simulink model "SEM_MBD_Bike_CMG_2017b"  (R2017b)
settings: Solver=FixedStepAuto  StartTime=0.0  StopTime=Tend  FixedStep=1e-3  MaxStep=0.01  RelTol=1e-4  AbsTol=1e-5  EnableMultiTasking=on
PreLoadFcn:
  | addpath(genpath('SM_Contact'))
  | addpath('include')
InitFcn:
  | MBD_Intfn
model workspace (MATLAB code in the model file):
  | whl.rad = 0.025;
  | whl.thickness = 0.005;
  | 
  | axle.length = 0.2;
  | axle.radius = 0.005;
  | platform.radius = 0.15;
  | platform.thickness = 0.005;
  | platform.offset = -0.01;
  | 
  | bumper.rad = platform.offset+whl.rad;
  | 
  | 
  | 
  | table.length = 1;
  | table.thickness = 0.01;
  | tableWhl.contact.k = 1e3;
  | tableWhl.contact.b = 1e2;
  | 
  | steel.density = 8000; %kg/m^3
  | 
  | start_pos.x = -0.2;
  | start_pos.y = 0.2;
  | 
  | l_whl_trq = [0 0 0 0.5 0 0 0 -0.5 1.0 0 0 0 -1.0 0.5 0 0 0 -0.5 -1.5 0 0 0 1.5].'*0.0005;
  | r_whl_trq = [0 0 0 2.0 0 0 0 -2.0 1.0 0 0 0 -1.0 1.0 0 0 0 -1.0 -1.5 0 0 0 1.5].'*0.0005;
values from neighbouring files (symbols this model uses):
  Dfw = 0.6    [MBD_Intfn.m]
  Drw = 0.6    [MBD_Intfn.m]
  followerCameraX = -1.5    [MBD_Intfn.m]
  followerCameraY = 0.5    [MBD_Intfn.m]
  followerCameraZ = -3    [MBD_Intfn.m]
  H = 1/2    (= 0.5)    [MBD_Intfn.m]
  IntG = 70    [MBD_Intfn.m]
  IntP = 0    [MBD_Intfn.m]
  isoCameraAimX = (1/2)*L    (= 1)    [MBD_Intfn.m]
  isoCameraX = -3.1    [MBD_Intfn.m]
  isoCameraY = 3.5    [MBD_Intfn.m]
  isoCameraZ = 1.5    [MBD_Intfn.m]
  Kdelta = -2.5    [MBD_Intfn.m]
  Kdeltadot = -5    [MBD_Intfn.m]
  Kphi = -60    [MBD_Intfn.m]
  Kphidot = -6    [MBD_Intfn.m]
  Ktheta = 0.1    [MBD_Intfn.m]
  Kthetadot = -5    [MBD_Intfn.m]
  Kv = -2.69    [MBD_Intfn.m]
  L = 2    [MBD_Intfn.m]
  Ldelta = 15    [MBD_Intfn.m]
  M = 10    [MBD_Intfn.m]
  MF = 1    [MBD_Intfn.m]
  Mf = 2    [MBD_Intfn.m]
  MR = 1    [MBD_Intfn.m]
  Nf = 5000    [MBD_Intfn.m]
  Rdelta = 0    [MBD_Intfn.m]
  refphi = 0    [MBD_Intfn.m]
  reftheta = 0    [MBD_Intfn.m]
  Rf = 0.2    [MBD_Intfn.m]
  Switch = 0    [MBD_Intfn.m]
  T = 0.05    [MBD_Intfn.m]
  tdl = 10    [MBD_Intfn.m]
  tdr = 1    [MBD_Intfn.m]
  Tend = 35    [MBD_Intfn.m]
  Tf = 0.3/5    (= 0.06)    [MBD_Intfn.m]
  topCameraX = -4.5    [MBD_Intfn.m]
  topCameraY = 0    [MBD_Intfn.m]
  topCameraZ = -0.5    [MBD_Intfn.m]
  tpdl = 10    [MBD_Intfn.m]
  tpdr = 1    [MBD_Intfn.m]
  v = 5    [MBD_Intfn.m]
undefined symbols (not defined in the file or in its folder): Floor, X, Y, Z
libraries: sm_lib x52, nesl_utility x41, Parts_Lib x4, Contact_Forces_Lib x4, simulink x2, fl_lib x1
(part 1 of 3)
Description:
  | A simulator for a simplified bicycle model including a CMG
  | 
  | By:
  | Dinesh Thirumurugan
  | Bhavesh Kataria
  | Allauddin Shaikh
  | Alen Turnwald
settings Model: Creator=smiller  LastModifiedBy=Alen
settings SolverCC: PositivePriorityOrder=on  AutoInsertRateTranBlk=on
settings DataIOCC: MaxDataPoints=15000  SaveFormat=Array  SignalLoggingName=logsout_Robot_2_Whl
settings OptimizationCC: EnhancedBackFolding=on  PassReuseOutputArgsThreshold=0  MaxStackSize=64  OptimizeBlockOrder=speed  DifferentSizesBufferReuse=on
settings DebuggingCC: SolverPrmCheckMsg=warning  ParameterTunabilityLossMsg=error  UnconnectedInputMsg=none  UnconnectedOutputMsg=none  AllowSymbolicDim=off  SFUnexpectedBacktrackingDiag=warning  SFNoUnconditionalDefaultTransitionDiag=warning  SFExecutionAtInitializationDiag=none
settings HardwareCC: ProdBitPerPointer=32  ProdBitPerSizeT=32  ProdBitPerPtrDiffT=32  ProdLargestAtomicInteger=Long  ProdLargestAtomicFloat=Double  ProdWordSize=32  ProdHWDeviceType=ARM Compatible->ARM Cortex  UseEmbeddedCoderFeatures=off
settings ModelReferenceCC: PropagateSignalLabelsOutOfModel=off
settings SFSimCC: MATLABDynamicMemAlloc=off
settings RTWCC: SystemTargetFile=ert.tlc  HardwareBoard=Raspberry Pi  TemplateMakefile=ert_default_tmf  GenerateReport=on  Toolchain=GNU GCC Raspberry Pi  BuildConfiguration=Faster Runs  LaunchReport=on
settings CodeAppCC: ForceParamTrailComments=on  OperatorAnnotations=on
settings ERTTargetCC: ERTCustomFileBanners=off  SupportContinuousTime=on  SupportNonInlinedSFcns=on  RemoveResetFunc=off  SupportVariableSizeSignals=on  ModelStepFunctionPrototypeControlCompliant=off
settings ConfigComp: CovMetricSettings=dw  CovHtmlReporting=on  CovSaveCumulativeToWorkspaceVar=on  CovSaveSingleToWorkspaceVar=on  CovExternalEMLEnable=off  CovSFcnEnable=off
settings SimscapeCC: SimscapeNormalizeSystem=off  SimscapeLogType=all  SimscapeLogSimulationStatistics=on  SimscapeLogName=simlog_Robot_2_Whl  SimscapeLogDataHistory=15000
settings ConfigurationSet: Description=SimMechanics 2G
settings DiagnosticsConfigSet: SimMechanicsRigidlyBoundBlock=none
settings ExplorerConfigSet: InternalSimMechanicsExplorerSettings="<ExplorerConfiguration><canonicalview>default</canonicalview><AnimationSetting><BasePlaybackSpeed>1.0</BasePlaybackSpeed><PlaybackSpeedFactor>1.0</PlaybackSpeedFactor></AnimationSetting><TilePanel><TileInfo><Tiles Columns=\"2\" Count=\"2\" Rows=\"1\"><Column Weight=\"0.5\"/><Column Weight=\"0.5\"/><Row Weight=\"1\"/><Tile Height=\"1\" Width=\"1\" X=\"0\" Y=\"0\"/><Tile Height=\"1\" Width=\"1\" X=\"1\" Y=\"0\"/></Tiles></TileInfo><SceneInfo><SceneViewer><BGColor><R>0.913725495338439941</R><G>0.952941179275512695</G><B>0.952941179275512695</B></BGColor><Camera><DoPerspective>on</DoPerspective><Position><X>19.7957692472944586</X><Y>-22.1490524136403373</Y><Z>1.79876643323261254</Z></Position><Center><X>22.8384549439588795</X><Y>-22.2465600466053246</Y><Z>0.30459240962381362</Z></Center><Up><X>0</X><Y>0</Y><Z>1</Z></Up><ViewLimDist>1</ViewLimDist><YLim>0.466307658154998583</YLim><XLim>0.393531318442946809</XLim></Camera></SceneViewer><SceneViewer><BGColor><R>0.913725495338439941</R><G>0.952941179275512695</G><B>0.952941179275512695</B></BGColor><Camera><DoPerspective>on</DoPerspective><Position><X>22.3361107324775219</X><Y>-22.2651355831809319</Y><Z>4.80429298217662559</Z></Position><Center><X>22.8384549439588795</X><Y>-22.2465600466053246</Y><Z>0.30459240962381362</Z></Center><Up><X>0</X><Y>0</Y><Z>1</Z></Up><ViewLimDist>1</ViewLimDist><YLim>0.466307658154998583</YLim><XLim>0.393531318442946809</XLim></Camera></SceneViewer></SceneInfo></TilePanel><MechEditorPanel><Cameras><Camera><Id>Camera1</Id><Value><Name>Follower Camera</Name><NativeCamera><PositionTrackingFeature>x1.Frame.Cameras.Follower_Camera_Transform.F</PositionTrackingFeature><CenterTrackingFeature>x1.Frame.Frame.R</CenterTrackingFeature><UpVectorTrackingFeature>x1.World_Frame.W</UpVectorTrackingFeature><CenterTrackingOrigin>on</CenterTrackingOrigin><UpVectorTrackingDirection>+Z</UpVectorTrackingDirection></NativeCamera></Value></Camera><Camera><Id>Camera2</Id><Value><Name>Top Camera</Name><NativeCamera><PositionTrackingFeature>x1.Frame.Cameras.Follower_Camera_Transform1.F</PositionTrackingFeature><CenterTrackingFeature>x1.Frame.Frame.R</CenterTrackingFeature><UpVectorTrackingFeature>x1.World_Frame.W</UpVectorTrackingFeature><CenterTrackingOrigin>on</CenterTrackingOrigin><UpVectorTrackingDirection>+Z</UpVectorTrackingDirection></NativeCamera></Value></Camera></Cameras><GfxPanelCameraMap><MapElement CameraMLId=\"Camera1\" GfxPanelIndex=\"0\"/><MapElement CameraMLId=\"Camera2\" GfxPanelIndex=\"1\"/></GfxPanelCameraMap><VideoCreator><PlaybackSpeedRatio>1.0</PlaybackSpeedRatio><FrameRate>30</FrameRate><VideoFormat>Motion JPEG AVI</VideoFormat><FrameSize>[800 600]</FrameSize></VideoCreator></MechEditorPanel></ExplorerConfiguration>"

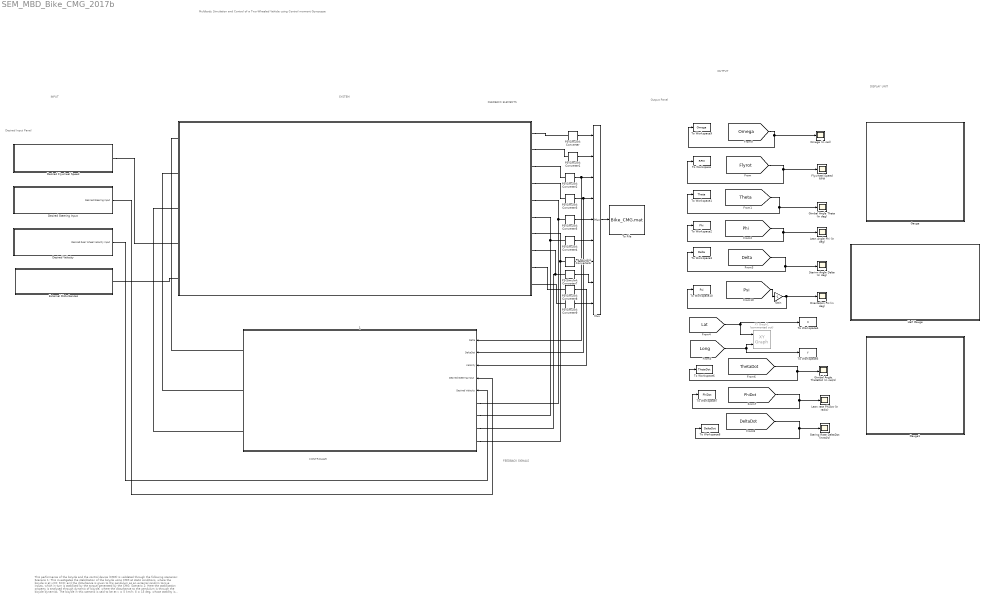
== system SEM_MBD_Bike_CMG_2017b ==
  note: Multibody Simulation and Control of a Two-Wheeled Vehicle using Control moment Gyroscope
  note: This performance of the bicycle and the control device (CMG) is validated through the following scenarios:
      |
      | Scenario 1: This investigates the stabilization of the bicycle using CMG at static conditions, where the bicycle is at v=0; δ=0; and the disturbance is given to the pendulum as an external random torque inputs, which in turn is stabilized by the torque generated by the CMG.
      |
      | Scenario 2: Here the stabilization property is analysed through dynamic of bicycle, where the disturbance to the pendulum is through the bicycle dynamics. The bicycle in this scenario is said to be at v = 5 km/h; δ = 15 deg, whose stability is analysed through the inverted pendulum which in turn is stabilized by the CMG.
      |
      | Scenario 3: The general behaviour of the bicycle dynamics is investigated in this scenario, here the control device is kept completely inactive and the pendulum is put at completely downward resting position. The bicycle is give a velocity v>0; and steering δ>0 for a specific time period to inspect the forces generated while cornering to produce a leaning behaviour by the pendulum approximating to that of the bicycle behaviour.
  note: Output Panel
  note: INPUT
  note: Desired Input Panel
  note: SYSTEM
  note: OUTPUT
  note: FEEDBACK SIGNALS
  note: CONTROLLER
  note: FEEDBACK ELEMENTS
  note: DISPLAY UNIT
  " " : Subsystem  mask(Controllers Parameters){Kphi=Kphi, Kphidot=Kphidot, Ktheta=Ktheta, Kthetadot=Kthetadot, refphi=refphi, reftheta=reftheta, Kdelta=Kdelta, Kdeltadot=Kdeltadot, Kv=Kv}
      mask prompts: Kphi "Proportional Gain Kφ"; Kphidot "Derivative Gain Kφ'"; Ktheta "Proptional Gain Kθ"; Kthetadot "Derivative Gain Kθ'"; refphi "Reference angle for pendulum (in deg)"; reftheta "Referance gimbal precision angle"; Kdelta "Proportional Gain Kδ"; Kdeltadot "Derivative Gain Kδ'"; Kv "Proportional Gain Kv"
      mask help:
      | PD Controller for Bicycle Stability:
      |
      | τ(θ) = −Kφ*(φ − φd) − Kφ˙*(φ˙) − Kθ*(θ − θd) − K˙θ*(˙θ).
      |
      | --------------------------------------------------------------------------------------------------------------------------------------------------------------
      | PD Controller for Steering:
      |
      | τ(δ) = −Kδ*(δ − δd) − K˙δ*(˙δ)
      |
      | --------------------------------------------------------------------------------------------------------------------------------------------------------------
      | PD Controller for Rear Wheel Torque:
      |
      | τ(v) = −Kv*(v − vd)
      mask Display: image('RPI.png')
  " 1" : Subsystem  mask(Controllers Parameters){Kphi=Kphi, Kphidot=Kphidot, Ktheta=Ktheta, Kthetadot=Kthetadot, refphi=refphi, reftheta=reftheta, Kdelta=Kdelta, Kdeltadot=Kdeltadot, Kv=Kv}
      mask prompts: Kphi "Proportional Gain Kφ"; Kphidot "Derivative Gain Kφ'"; Ktheta "Proptional Gain Kθ"; Kthetadot "Derivative Gain Kθ'"; refphi "Reference angle for pendulum (in deg)"; reftheta "Referance gimbal precision angle"; Kdelta "Proportional Gain Kδ"; Kdeltadot "Derivative Gain Kδ'"; Kv "Proportional Gain Kv"
      mask help:
      | PD Controller for Bicycle Stability:
      |
      | τ(θ) = −Kφ*(φ − φd) − Kφ˙*(φ˙) − Kθ*(θ − θd) − K˙θ*(˙θ).
      |
      | --------------------------------------------------------------------------------------------------------------------------------------------------------------
      | PD Controller for Steering:
      |
      | τ(δ) = −Kδ*(δ − δd) − K˙δ*(˙δ)
      |
      | --------------------------------------------------------------------------------------------------------------------------------------------------------------
      | PD Controller for Rear Wheel Torque:
      |
      | τ(v) = −Kv*(v − vd)
      mask Display: image('RPI.png')
  "           " : Subsystem  mask(Parameters of bicycle with CMG){cyl_dia_R=Drw, cyl_dia_F=Dfw, cyl_thickness=T, cyl_mass_R=MR, cyl_mass_F=MF, BaseL=L, Bikemass=M, Fly_R=Rf, Fly_T=Tf, Fly_M=Mf, CMG_H=H, IntP=IntP, IntG=IntG}
      mask prompts: cyl_dia_R "Diameter of rear wheel (in m)"; cyl_dia_F "Diameter of front wheel (in m)"; cyl_thickness "Wheel thickness (in m)"; cyl_mass_R "Mass of the rear wheel (in kg)"; cyl_mass_F "Mass of the front wheel (in kg)"; BaseL "Wheelbase (in m)"; Bikemass "Mass of the bicycle (frame included) (in kg)"; Fly_R "Radius of flywheel (in m)"; Fly_T "Thickness of flywheel (in m)"; Fly_M "Mass of flywheel (in kg)"; CMG_H "Height of the CMG (in m)"; IntP "Initial position of pendulum (in deg)"; IntG "Initial position of the gimbal (in deg)"
      mask help:
      | The given parameters are used for model creation.
      |
      | ------------------------------------------------------------------------------------------------------------------------------------------------------------------
      mask Display: image('Bike_CSs.jpg')
  Desired Flywheel Speed : Subsystem  mask(Flywheel Rotation Speed){w=Nf}
      mask prompts: w "Flywheel Speed (RPM)"
      mask help: Omega (RPM)
  Desired Steering Input : Subsystem  mask(Desired Steering Input){t=Tend, delta_L=Ldelta, l_t=tpdl, Lt=tdl, delta_R=Rdelta, r_t=tpdr, Rt=tdr}
      mask prompts: t "Total Time Duration (in sec)"; delta_L "Left Steering Angle (in deg)"; l_t "Phase delay - Left Steering (in sec)"; Lt "Duration for Left Steering (in sec)"; delta_R "Right Steering Angle (in deg)"; r_t "Phase delay - Right Steering (in sec)"; Rt "Duration for Right Steering (in sec)"
      mask help:
      | This block helps to build a steering profile for the bicycle to follow.
      |
      | --------------------------------------------------------------------------------------------------------------------------------------------------------------
      | Total Time Duration  = Total time duration for simulation signal (in sec)
      |
      | %Left steering inputs
      | Left Steering Angle (in deg) = Left steering angle (in deg) defines the angle input requried for left steering
      | Phase delay - Left Steering (in sec) = Phase delay for left steering (in sec) defines the time duration after which the left steering angle input should be achived
      | Duration for Left Steering (in sec) = Duration for the left steering (in sec) defines the duration for which the left steering signal should be active
      |
      | %Right steering inputs
      | Right Steering Angle (in deg) = Right steering angle (in deg) defines the angle input requried for right steering
      | Phase delay - Right Steering (in sec) = Phase delay for right steering (in sec) defines the time duration after which the right steering angle input should be achived
      | Duration for Right Steering (in sec) = Duration for the right steering (in sec) defines the duration for which the right steering signal should be active
  Desired Velocity : Subsystem  mask{v=v}
      mask prompts: v "Desired Velocity (kmph)"
  External Disturbances : Subsystem  mask{Switch=Switch}
      mask prompts: Switch "External Disturbance Enable/Disable"
  Flywheel Speed RPM : Scope
  Gain : Gain  Gain=-1
  Gauge : Subsystem  DialogController=hmiCreateDDGDialog  IsWebBlock=on  mask(MWDashboardBlock){webBlockId=e0acaf17-1707-462e-bd3e-ad1907f2a35e, webBlockType=circulargauge, ShowInLibBrowser=on, ShowInitialText=on, HMISrcModelName=SEM_MBD_Bike_CMG_2017b}
      mask prompts: webBlockId "WebBlock Id"; webBlockType "WebBlock Type"; HMISrcModelName "Source Model"
      mask help: SimulinkHMI:dialogs:CircularGaugeDialogDesc
      mask Help: helpview([docroot '/mapfiles/simulink.map'], 'hmi_gauge')
      mask Display:
      | if strcmp(get_param(bdroot(gcb),'BlockDiagramType'), 'library')
      |     image([(matlabroot) '/toolbox/simulink/hmi/icons/CircularGauge.png']);
      | end
  Gauge1 : Subsystem  DialogController=hmiCreateDDGDialog  IsWebBlock=on  mask(MWDashboardBlock){webBlockId=d5ddcee6-ece7-4a8c-aff1-6e72436c5361, webBlockType=circulargauge, ShowInLibBrowser=on, ShowInitialText=on, HMISrcModelName=SEM_MBD_Bike_CMG_2017b}
      mask prompts: webBlockId "WebBlock Id"; webBlockType "WebBlock Type"; HMISrcModelName "Source Model"
      mask help: SimulinkHMI:dialogs:CircularGaugeDialogDesc
      mask Help: helpview([docroot '/mapfiles/simulink.map'], 'hmi_gauge')
      mask Display:
      | if strcmp(get_param(bdroot(gcb),'BlockDiagramType'), 'library')
      |     image([(matlabroot) '/toolbox/simulink/hmi/icons/CircularGauge.png']);
      | end
  Gimbal Angle Theta (in deg) : Scope
  Gimbal Angle ThetaDot (in rad/s) : Scope
  Half Gauge : Subsystem  DialogController=hmiCreateDDGDialog  IsWebBlock=on  mask(MWDashboardBlock){webBlockId=2bf35224-e477-42b1-a6f6-088c116ad7f4, webBlockType=semicirculargauge, ShowInLibBrowser=on, ShowInitialText=on, HMISrcModelName=SEM_MBD_Bike_CMG_2017b}
      mask prompts: webBlockId "WebBlock Id"; webBlockType "WebBlock Type"; HMISrcModelName "Source Model"
      mask help: SimulinkHMI:dialogs:SemicircularGaugeDialogDesc
      mask Help: helpview([docroot '/mapfiles/simulink.map'], 'hmi_half_gauge')
      mask Display:
      | if strcmp(get_param(bdroot(gcb),'BlockDiagramType'), 'library')
      |     image([(matlabroot) '/toolbox/simulink/hmi/icons/SemicircularGauge.png']);
      | end
  "Lean Angle Phi (in deg) " : Scope
  Lean rate PhiDot (in rad/s) : Scope
  Mux : Mux  Inputs=9
  Omega (in rad) : Scope
  Orientation Psi (in deg) : Scope
  PS-Simulink Converter : nesl_utility/PS-Simulink Converter  PhysicalDomain=network_engine_domain  SubClassName=ps_output  LeftPortType=input  RightPortType=output  PseudoPeriodic=off  Frequencies=[]  Unit=m  AffineConversion=off
  PS-Simulink Converter1 : nesl_utility/PS-Simulink Converter  PhysicalDomain=network_engine_domain  SubClassName=ps_output  LeftPortType=input  RightPortType=output  PseudoPeriodic=off  Frequencies=[]  Unit=m  AffineConversion=off
  PS-Simulink Converter{2..9} (8 alike) : nesl_utility/PS-Simulink Converter  PhysicalDomain=network_engine_domain  SubClassName=ps_output  LeftPortType=input  RightPortType=output  PseudoPeriodic=off  Frequencies=[]  Unit=1  AffineConversion=off
  Stering Angle Delta (in deg) : Scope
  Stering Rate DeltaDot (inrad/s) : Scope
  To File : ToFile  Filename=Bike_CMG.mat  MatrixName=output  SaveFormat=Timeseries
  To Workspace : ToWorkspace  VariableName=RPM  SaveFormat=Timeseries  SampleTime=-1
  To Workspace1 : ToWorkspace  VariableName=Theta  SaveFormat=Timeseries  SampleTime=-1
  To Workspace10 : ToWorkspace  VariableName=Psi  SaveFormat=Timeseries  SampleTime=-1
  To Workspace2 : ToWorkspace  VariableName=Phi  SaveFormat=Timeseries  SampleTime=-1
  To Workspace3 : ToWorkspace  VariableName=Delta  SaveFormat=Timeseries  SampleTime=-1
  To Workspace4 : ToWorkspace  VariableName=X  SaveFormat=Timeseries  SampleTime=-1
  To Workspace5 : ToWorkspace  VariableName=Y  SaveFormat=Timeseries  SampleTime=-1
  To Workspace6 : ToWorkspace  VariableName=ThetaDot  SaveFormat=Timeseries  SampleTime=-1
  To Workspace7 : ToWorkspace  VariableName=PhiDot  SaveFormat=Timeseries  SampleTime=-1
  To Workspace8 : ToWorkspace  VariableName=DeltaDot  SaveFormat=Timeseries  SampleTime=-1
  To Workspace9 : ToWorkspace  VariableName=Omega  SaveFormat=Timeseries  SampleTime=-1
  XY Graph1 : simulink/Sinks/XY Graph  Commented=on  xmin=-50  xmax=50  ymin=-50  ymax=50  st=0.5
  wires:
  [Flyrot] -> To Workspace/1, Flywheel Speed RPM/1
  [Theta] -> To Workspace1/1, Gimbal Angle Theta (in deg)/1
  [Phi] -> To Workspace2/1, "Lean Angle Phi (in deg) "/1
  [Delta] -> To Workspace3/1, Stering Angle Delta (in deg)/1
  [Lat] -> XY Graph1/1, To Workspace4/1
  [Long] -> XY Graph1/2, To Workspace5/1
  [ThetaDot] -> To Workspace6/1, Gimbal Angle ThetaDot (in rad/s)/1
  [PhiDot] -> To Workspace7/1, Lean rate PhiDot (in rad/s)/1
  [DeltaDot] -> To Workspace8/1, Stering Rate DeltaDot (inrad/s)/1
  PS-Simulink Converter7/1 -> Mux/8
  PS-Simulink Converter6/1 -> Mux/7
  PS-Simulink Converter4/1 -> Mux/6
  PS-Simulink Converter5/1 -> Mux/5
  PS-Simulink Converter1/1 -> Mux/2
  PS-Simulink Converter/1 -> Mux/1
  PS-Simulink Converter9/1 -> Mux/9
  Mux/1 -> To File/1
  PS-Simulink Converter2/1 -> " "/1(Delta), Mux/3
  PS-Simulink Converter8/1 -> " "/3(Velocity)
  PS-Simulink Converter3/1 -> " "/2(DeltaDot), Mux/4
  Desired Steering Input/1(Desired Steering Input) -> " "/4(Desired Steering Input)
  Desired Velocity/1(Desired Rear Wheel Velocity Input) -> " "/5(Desired Velocity)
  [Omega] -> To Workspace9/1, Omega (in rad)/1
  [Psi] -> Gain/1
  Gain/1 -> To Workspace10/1, Orientation Psi (in deg)/1
  connections:
  "           "/LConn1 -- PS-Simulink Converter/LConn1
  "           "/LConn2 -- PS-Simulink Converter1/LConn1
  "           "/LConn3 -- PS-Simulink Converter2/LConn1
  "           "/LConn4 -- PS-Simulink Converter3/LConn1
  "           "/LConn5 -- " "/LConn1 -- PS-Simulink Converter5/LConn1
  "           "/LConn6 -- " "/LConn2 -- PS-Simulink Converter4/LConn1
  "           "/LConn7 -- " "/LConn4 -- PS-Simulink Converter6/LConn1
  "           "/LConn8 -- " "/LConn3 -- PS-Simulink Converter7/LConn1
  "           "/LConn9 -- PS-Simulink Converter8/LConn1
  " "/RConn1 -- "           "/RConn1
  " "/RConn2 -- "           "/RConn2
  " "/RConn3 -- "           "/RConn3
  PS-Simulink Converter9/LConn1 -- "           "/LConn10
  Desired Flywheel Speed/RConn1 -- "           "/RConn4
  "           "/RConn5 -- External Disturbances/RConn1

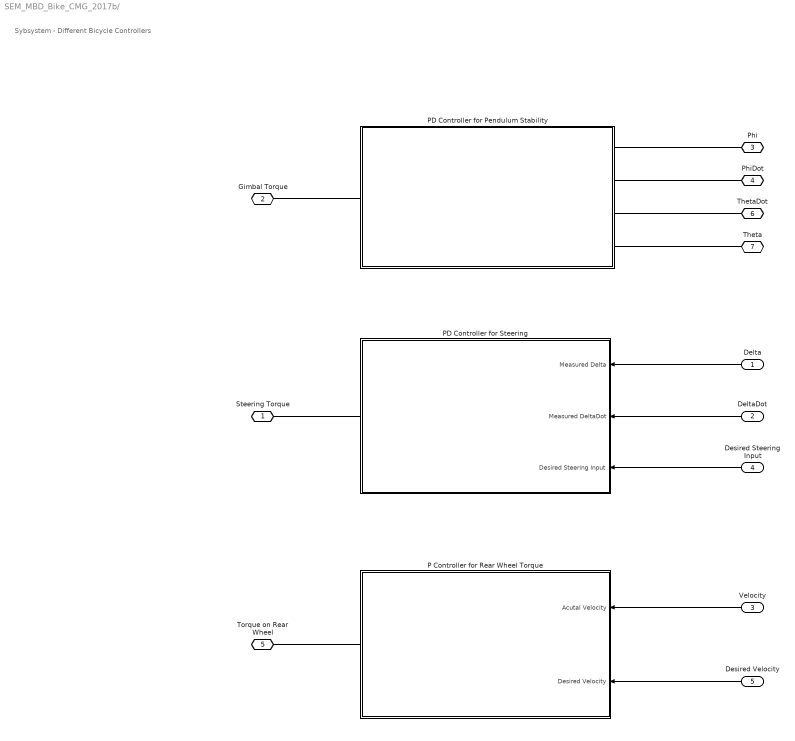
== system SEM_MBD_Bike_CMG_2017b/  ==
  note: Sybsystem - Different Bicycle Controllers
  Delta : Inport
  DeltaDot : Inport  Port=2
  Velocity : Inport  Port=3
  Desired Steering Input : Inport  Port=4
  Desired Velocity : Inport  Port=5
  "P Controller for Rear Wheel Torque " : Subsystem
  "PD Controller for Pendulum Stability " : Subsystem
  "PD Controller for Steering " : Subsystem
  Steering Torque : PMIOPort  Port=1  Side=Right
  "Gimbal Torque " : PMIOPort  Port=2  Side=Right
  Phi : PMIOPort  Port=3  Side=Left
  PhiDot : PMIOPort  Port=4  Side=Left
  Torque on Rear Wheel : PMIOPort  Port=5  Side=Right
  ThetaDot : PMIOPort  Port=6  Side=Left
  Theta : PMIOPort  Port=7  Side=Left
  wires:
  Delta/1 -> "PD Controller for Steering "/1(Measured Delta)
  Velocity/1 -> "P Controller for Rear Wheel Torque "/1(Acutal Velocity)
  DeltaDot/1 -> "PD Controller for Steering "/2(Measured DeltaDot)
  Desired Steering Input/1 -> "PD Controller for Steering "/3(Desired Steering Input)
  Desired Velocity/1 -> "P Controller for Rear Wheel Torque "/2(Desired Velocity)
  connections:
  "PD Controller for Pendulum Stability "/LConn1 -- Phi/RConn1
  "P Controller for Rear Wheel Torque "/RConn1 -- Torque on Rear Wheel/RConn1
  "PD Controller for Pendulum Stability "/LConn2 -- PhiDot/RConn1
  "PD Controller for Pendulum Stability "/LConn3 -- ThetaDot/RConn1
  "PD Controller for Steering "/RConn1 -- Steering Torque/RConn1
  "PD Controller for Pendulum Stability "/RConn1 -- "Gimbal Torque "/RConn1
  Theta/RConn1 -- "PD Controller for Pendulum Stability "/LConn4

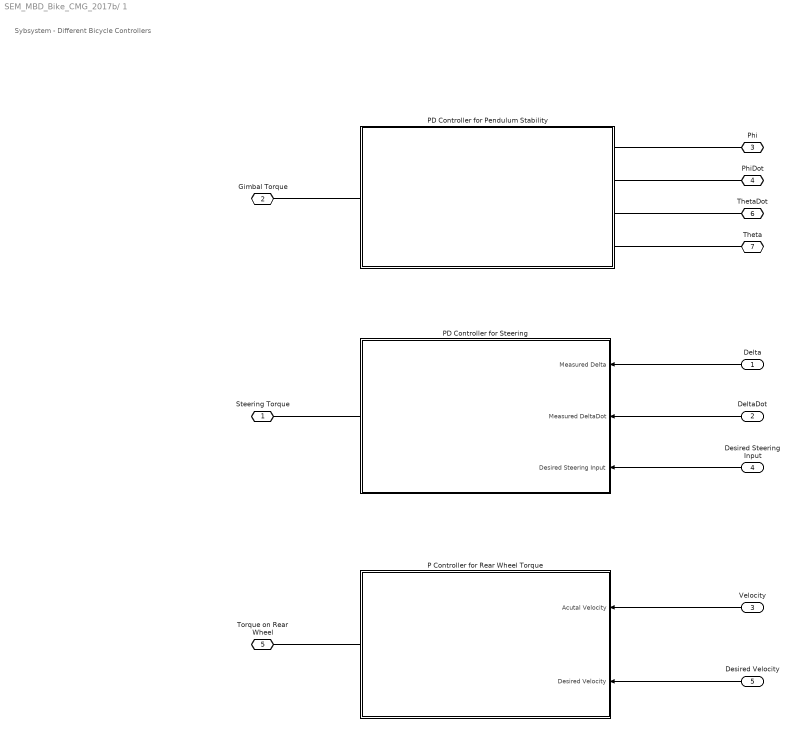
== system SEM_MBD_Bike_CMG_2017b/ 1 ==
  note: Sybsystem - Different Bicycle Controllers
  Delta : Inport
  DeltaDot : Inport  Port=2
  Velocity : Inport  Port=3
  Desired Steering Input : Inport  Port=4
  Desired Velocity : Inport  Port=5
  "P Controller for Rear Wheel Torque " : Subsystem
  "PD Controller for Pendulum Stability " : Subsystem
  "PD Controller for Steering " : Subsystem
  Steering Torque : PMIOPort  Port=1  Side=Right
  "Gimbal Torque " : PMIOPort  Port=2  Side=Right
  Phi : PMIOPort  Port=3  Side=Left
  PhiDot : PMIOPort  Port=4  Side=Left
  Torque on Rear Wheel : PMIOPort  Port=5  Side=Right
  ThetaDot : PMIOPort  Port=6  Side=Left
  Theta : PMIOPort  Port=7  Side=Left
  wires:
  Desired Velocity/1 -> "P Controller for Rear Wheel Torque "/2(Desired Velocity)
  Desired Steering Input/1 -> "PD Controller for Steering "/3(Desired Steering Input)
  DeltaDot/1 -> "PD Controller for Steering "/2(Measured DeltaDot)
  Velocity/1 -> "P Controller for Rear Wheel Torque "/1(Acutal Velocity)
  Delta/1 -> "PD Controller for Steering "/1(Measured Delta)
  connections:
  Theta/RConn1 -- "PD Controller for Pendulum Stability "/LConn4
  "PD Controller for Pendulum Stability "/RConn1 -- "Gimbal Torque "/RConn1
  "PD Controller for Steering "/RConn1 -- Steering Torque/RConn1
  "PD Controller for Pendulum Stability "/LConn3 -- ThetaDot/RConn1
  "PD Controller for Pendulum Stability "/LConn2 -- PhiDot/RConn1
  "P Controller for Rear Wheel Torque "/RConn1 -- Torque on Rear Wheel/RConn1
  "PD Controller for Pendulum Stability "/LConn1 -- Phi/RConn1

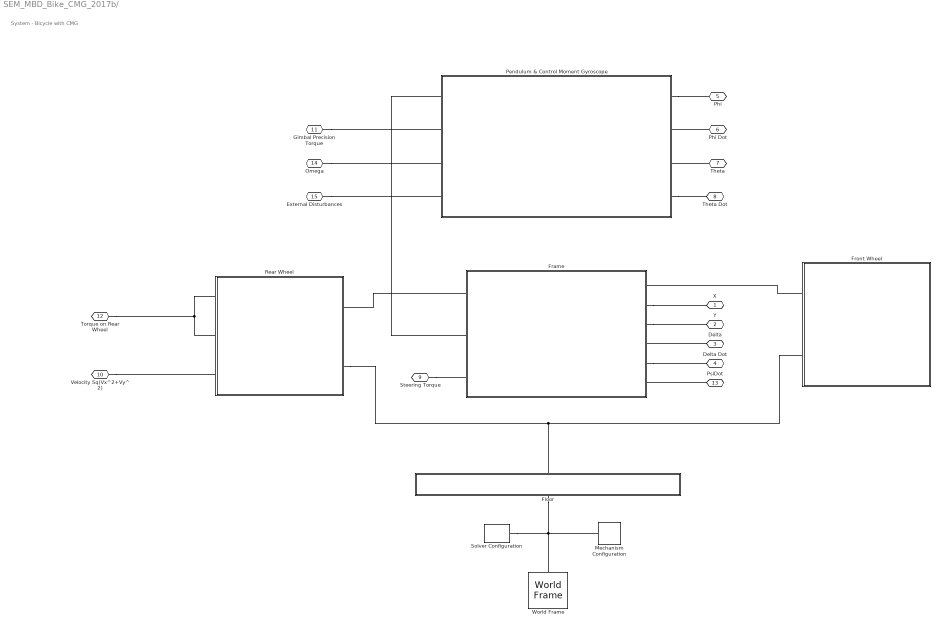
== system SEM_MBD_Bike_CMG_2017b/            ==
  note: System - Bicycle with CMG
  "  Floor" : Subsystem  Tag=CustomStyle
  " World Frame " : sm_lib/Frames and Transforms/World Frame
  "Frame " : Subsystem
      mask Display: image('Frame.png');
  "Front Wheel " : Subsystem
      mask Display: image('Front Wheel.png');
  Mechanism Configuration : sm_lib/Utilities/Mechanism Configuration  UniformGravity=Constant  GravityVector=[0 0 -9.80665]  GravityUnits=m/s^2  LinearizationDelta=0.001
  "Pendulum & Control Moment Gyroscope " : Subsystem
      mask Display: image('Pendulum_1.JPG');
  "Rear Wheel " : Subsystem
      mask Display: image('Rear Wheel.png');
  Solver Configuration : nesl_utility/Solver Configuration  PhysicalDomain=network_engine_domain  SubClassName=solver  LeftPortType=input  RightPortType=generic  Accelerate=off  Tones=[]  Harmonics=[]  SimulateNoise=off  Profile=off  UseLocalSampling=off  EnableSwitchedLinearOptims=on  FrequencyDomain=off  UseCCode=off  RelTol=0.001  AbsTol=1e-06  MinStep=1e-09  ToWorkspace=off  RevertToSquareIcSolve=off  NumHomotopyIterations=100  PhasorMode=off  PhasorModeNumHarmonics=1  DoDC=off  ResidualTolerance=1e-09  UseLocalSolver=off  LocalSolverChoice=NE_BACKWARD_EULER_ADVANCER  LocalSolverSampleTime=0.001  DoFixedCost=off  MaxNonlinIter=3  MaxModeIter=2  LinearAlgebra=Sparse  DelaysMemoryBudget=1024  AutomaticFiltering=on  FilteringTimeConstant=0.000001
  X : PMIOPort  Port=1  Side=Left
  Y : PMIOPort  Port=2  Side=Left
  Delta : PMIOPort  Port=3  Side=Left
  Delta Dot : PMIOPort  Port=4  Side=Left
  Phi : PMIOPort  Port=5  Side=Left
  Phi Dot : PMIOPort  Port=6  Side=Left
  "Theta " : PMIOPort  Port=7  Side=Left
  Theta Dot : PMIOPort  Port=8  Side=Left
  "Steering Torque " : PMIOPort  Port=9  Side=Right
  Velocity Sq(Vx^2+Vy^2) : PMIOPort  Port=10  Side=Left
  Gimbal Precision Torque : PMIOPort  Port=11  Side=Right
  Torque on Rear Wheel : PMIOPort  Port=12  Side=Right
  " PsiDot" : PMIOPort  Port=13  Side=Left
  Omega : PMIOPort  Port=14  Side=Right
  External Disturbances : PMIOPort  Port=15  Side=Right
  connections:
  "Frame "/LConn1 -- "Rear Wheel "/RConn1
  "Front Wheel "/LConn1 -- "Frame "/RConn1
  "Front Wheel "/LConn2 -- "Rear Wheel "/RConn2 -- "  Floor"/LConn1
  "Pendulum & Control Moment Gyroscope "/LConn1 -- "Frame "/LConn2
  "  Floor"/RConn1 -- Mechanism Configuration/RConn1 -- Solver Configuration/RConn1 -- " World Frame "/RConn1
  "Steering Torque "/RConn1 -- "Frame "/LConn3
  Gimbal Precision Torque/RConn1 -- "Pendulum & Control Moment Gyroscope "/LConn2
  Torque on Rear Wheel/RConn1 -- "Rear Wheel "/LConn2 -- "Rear Wheel "/LConn1
  "Frame "/RConn2 -- X/RConn1
  "Frame "/RConn3 -- Y/RConn1
  "Pendulum & Control Moment Gyroscope "/RConn1 -- Phi/RConn1
  Phi Dot/RConn1 -- "Pendulum & Control Moment Gyroscope "/RConn2
  Delta/RConn1 -- "Frame "/RConn4
  "Frame "/RConn5 -- Delta Dot/RConn1
  "Theta "/RConn1 -- "Pendulum & Control Moment Gyroscope "/RConn3
  "Pendulum & Control Moment Gyroscope "/RConn4 -- Theta Dot/RConn1
  Velocity Sq(Vx^2+Vy^2)/RConn1 -- "Rear Wheel "/LConn3
  " PsiDot"/RConn1 -- "Frame "/RConn6
  Omega/RConn1 -- "Pendulum & Control Moment Gyroscope "/LConn3
  External Disturbances/RConn1 -- "Pendulum & Control Moment Gyroscope "/LConn4

== system SEM_MBD_Bike_CMG_2017b/Desired Flywheel Speed ==
  note: Subsystem - Desired Flywheel Speed with Unit Conversions
  Fkywheel Speed RPM : Constant  Value=w
  "Integrator " : Integrator
  "Signal Specification " : SignalSpecification  Unit=rpm
  Signal Specification (rpm-rad/s) : SignalSpecification  Unit=rad/s
  Simulink-PS Converter : nesl_utility/Simulink-PS Converter  PhysicalDomain=network_engine_domain  SubClassName=ps_input  LeftPortType=input  RightPortType=output  PseudoPeriodic=off  Frequencies=[]  NoiseDistribution=none  NoiseParameters=[]  Unit=rad  AffineConversion=off  FilteringAndDerivatives=filter  SimscapeFilterOrder=2  InputFilterTimeConstant=1  UdotUserProvided=0
  "Unit Conversion " : UnitConversion
  Flywheel Speed : PMIOPort  Port=1  Side=Right
  wires:
  "Integrator "/1 -> Simulink-PS Converter/1
  "Signal Specification "/1 -> "Unit Conversion "/1
  Signal Specification (rpm-rad/s)/1 -> "Integrator "/1
  "Unit Conversion "/1 -> Signal Specification (rpm-rad/s)/1
  Fkywheel Speed RPM/1 -> "Signal Specification "/1
  connections:
  Simulink-PS Converter/RConn1 -- Flywheel Speed/RConn1

== system SEM_MBD_Bike_CMG_2017b/Desired Steering Input ==
  note: Subsystem - Desired Steering Input
  Pulse Generator (Left Steering) : DiscretePulseGenerator  PulseType=Time based  Amplitude=delta_L  Period=Tend  PulseWidth=Lt*100/Tend  PhaseDelay=l_t
  "Pulse Generator (Right Steering) " : DiscretePulseGenerator  PulseType=Time based  Amplitude=delta_R  Period=Tend  PulseWidth=Rt*100/Tend  PhaseDelay=r_t
  Scope : Scope
  Scope1 : Scope
  Scope2 : Scope
  Sum1 : Sum  Inputs=+|-
  To Workspace : ToWorkspace  VariableName=DeltaDesired  SaveFormat=Timeseries  SampleTime=-1
  Unit Conversion (Deg - rad) : Gain  Gain=pi/180
  Desired Steering Input : Outport
  wires:
  "Pulse Generator (Right Steering) "/1 -> Sum1/1, Scope/1
  Sum1/1 -> To Workspace/1, Unit Conversion (Deg - rad)/1
  Unit Conversion (Deg - rad)/1 -> Scope2/1, Desired Steering Input/1
  Pulse Generator (Left Steering)/1 -> Scope1/1, Sum1/2

== system SEM_MBD_Bike_CMG_2017b/Desired Velocity ==
  note: Subsystem - Desired Bike Rear Wheel Velocity Input
  Bike Speed Kmph1 : Constant  Value=v
  Desired Rear Wheel Velocity Input : Outport
  wires:
  Bike Speed Kmph1/1 -> Desired Rear Wheel Velocity Input/1

== system SEM_MBD_Bike_CMG_2017b/External Disturbances ==
  note: Subsystem - External Disturbance Input
  Gain : Gain  Gain=Switch
  Random White Noise Disturbance : simulink/Sources/Band-Limited White Noise  Cov=[0.1]  Ts=0.1  seed=[23341]
  Rate Transition : RateTransition
  Scope : Scope
  Simulink-PS Converter : nesl_utility/Simulink-PS Converter  PhysicalDomain=network_engine_domain  SubClassName=ps_input  LeftPortType=input  RightPortType=output  PseudoPeriodic=off  Frequencies=[]  NoiseDistribution=none  NoiseParameters=[]  Unit=N*m  AffineConversion=off  FilteringAndDerivatives=provide  SimscapeFilterOrder=1  InputFilterTimeConstant=0.001  UdotUserProvided=0
  To Workspace : ToWorkspace  VariableName=U_ex  SaveFormat=Timeseries  SampleTime=-1
  External Disturbances : PMIOPort  Port=1  Side=Right
  wires:
  Random White Noise Disturbance/1 -> Rate Transition/1
  Gain/1 -> Simulink-PS Converter/1, Scope/1, To Workspace/1
  Rate Transition/1 -> Gain/1
  connections:
  Simulink-PS Converter/RConn1 -- External Disturbances/RConn1

== system SEM_MBD_Bike_CMG_2017b/Gauge ==

== system SEM_MBD_Bike_CMG_2017b/Gauge1 ==

== system SEM_MBD_Bike_CMG_2017b/Half Gauge ==

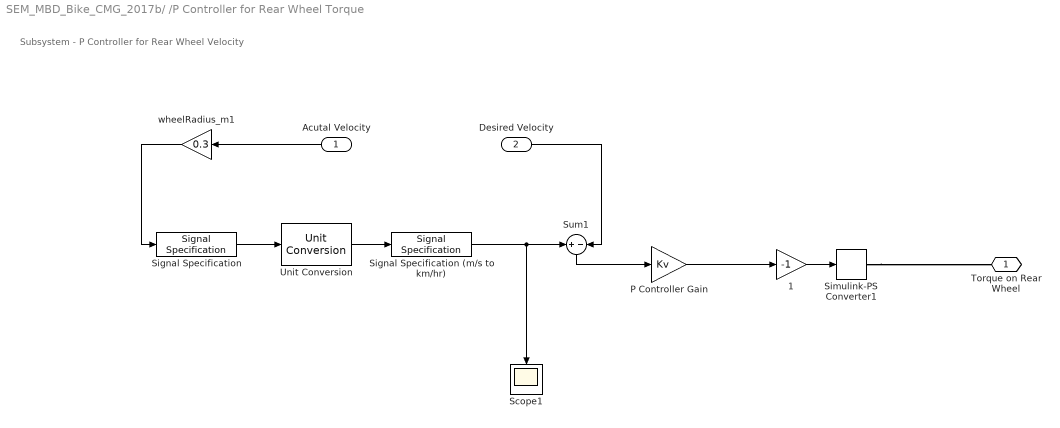
== system SEM_MBD_Bike_CMG_2017b/ /P Controller for Rear Wheel Torque  ==
  note: Subsystem - P Controller for Rear Wheel Velocity
  Acutal Velocity : Inport
  Desired Velocity : Inport  Port=2
  1 : Gain  Gain=-1
  P Controller Gain : Gain  Gain=Kv
  Scope1 : Scope
  "Signal Specification " : SignalSpecification  Unit=m/s
  Signal Specification (m/s to km/hr) : SignalSpecification  Unit=km/hr
  Simulink-PS Converter1 : nesl_utility/Simulink-PS Converter  PhysicalDomain=network_engine_domain  SubClassName=ps_input  LeftPortType=input  RightPortType=output  PseudoPeriodic=off  Frequencies=[]  NoiseDistribution=none  NoiseParameters=[]  Unit=N*m  AffineConversion=off  FilteringAndDerivatives=filter  SimscapeFilterOrder=2  InputFilterTimeConstant=1  UdotUserProvided=0
  Sum1 : Sum  Inputs=+|-
  "Unit Conversion " : UnitConversion
  wheelRadius_m1 : Gain  Gain=0.3
      settings: AttributesFormatString=%<Gain>
  Torque on Rear Wheel : PMIOPort  Port=1  Side=Right
  wires:
  wheelRadius_m1/1 -> "Signal Specification "/1
  "Signal Specification "/1 -> "Unit Conversion "/1
  Sum1/1 -> P Controller Gain/1
  Signal Specification (m/s to km/hr)/1 -> Sum1/1, Scope1/1
  P Controller Gain/1 -> 1/1
  "Unit Conversion "/1 -> Signal Specification (m/s to km/hr)/1
  Acutal Velocity/1 -> wheelRadius_m1/1
  1/1 -> Simulink-PS Converter1/1
  Desired Velocity/1 -> Sum1/2
  connections:
  Simulink-PS Converter1/RConn1 -- Torque on Rear Wheel/RConn1

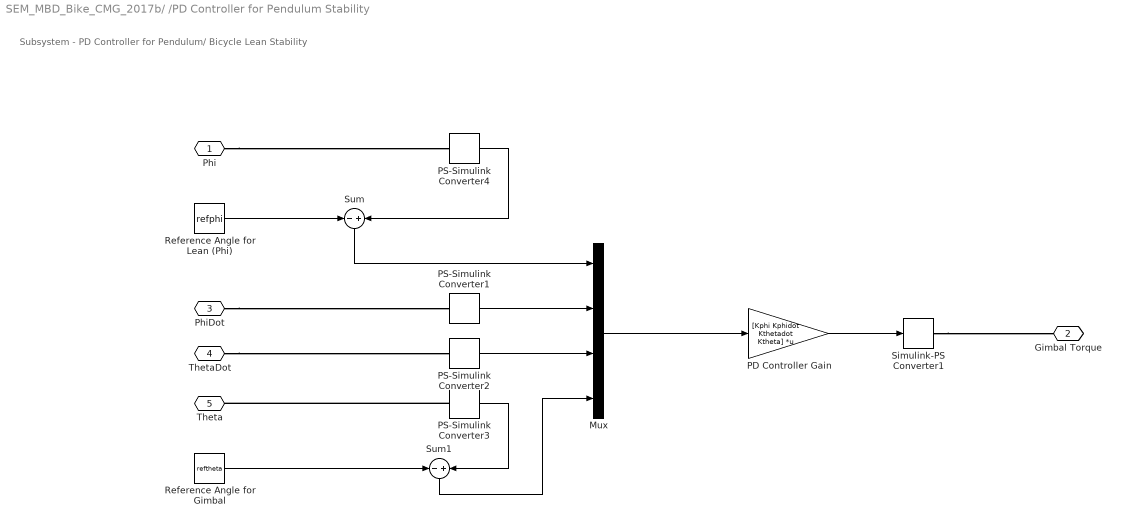
== system SEM_MBD_Bike_CMG_2017b/ /PD Controller for Pendulum Stability  ==
  note: Subsystem - PD Controller for Pendulum/ Bicycle Lean Stability
  Mux : Mux
  PD Controller Gain : Gain  Gain=[Kphi Kphidot Kthetadot Ktheta]  Multiplication=Matrix(K*u)
  PS-Simulink Converter{1..4} (4 alike) : nesl_utility/PS-Simulink Converter  PhysicalDomain=network_engine_domain  SubClassName=ps_output  LeftPortType=input  RightPortType=output  PseudoPeriodic=off  Frequencies=[]  Unit=1  AffineConversion=off
  Reference Angle for Gimbal : Constant  Value=reftheta
  Reference Angle for Lean (Phi) : Constant  Value=refphi
  Simulink-PS Converter1 : nesl_utility/Simulink-PS Converter  PhysicalDomain=network_engine_domain  SubClassName=ps_input  LeftPortType=input  RightPortType=output  PseudoPeriodic=off  Frequencies=[]  NoiseDistribution=none  NoiseParameters=[]  Unit=N*m  AffineConversion=off  FilteringAndDerivatives=provide  SimscapeFilterOrder=1  InputFilterTimeConstant=0.001  UdotUserProvided=0
  Sum : Sum  Inputs=-|+
      settings: AttributesFormatString=Error
  Sum1 : Sum  Inputs=-|+
      settings: AttributesFormatString=Error
  Phi : PMIOPort  Port=1  Side=Left
  Gimbal Torque : PMIOPort  Port=2  Side=Right
  PhiDot : PMIOPort  Port=3  Side=Left
  ThetaDot : PMIOPort  Port=4  Side=Left
  Theta : PMIOPort  Port=5  Side=Left
  wires:
  Reference Angle for Lean (Phi)/1 -> Sum/1
  Sum/1 -> Mux/1
  PS-Simulink Converter1/1 -> Mux/2
  Mux/1 -> PD Controller Gain/1
  PD Controller Gain/1 -> Simulink-PS Converter1/1
  PS-Simulink Converter2/1 -> Mux/3
  Reference Angle for Gimbal/1 -> Sum1/1
  PS-Simulink Converter3/1 -> Sum1/2
  Sum1/1 -> Mux/4
  PS-Simulink Converter4/1 -> Sum/2
  connections:
  Phi/RConn1 -- PS-Simulink Converter4/LConn1
  PhiDot/RConn1 -- PS-Simulink Converter1/LConn1
  ThetaDot/RConn1 -- PS-Simulink Converter2/LConn1
  Simulink-PS Converter1/RConn1 -- Gimbal Torque/RConn1
  PS-Simulink Converter3/LConn1 -- Theta/RConn1

== system SEM_MBD_Bike_CMG_2017b/ /PD Controller for Steering  ==
  note: Subsystem - PD Controller for Bicycle Steering
  Measured Delta : Inport
  Measured DeltaDot : Inport  Port=2
  Desired Steering Input : Inport  Port=3
  Mux : Mux  Inputs=2
  PD Controller Gain : Gain  Gain=[Kdelta Kdeltadot]  Multiplication=Matrix(K*u)
  Simulink-PS Converter : nesl_utility/Simulink-PS Converter  PhysicalDomain=network_engine_domain  SubClassName=ps_input  LeftPortType=input  RightPortType=output  PseudoPeriodic=off  Frequencies=[]  NoiseDistribution=none  NoiseParameters=[]  Unit=1  AffineConversion=off  FilteringAndDerivatives=provide  SimscapeFilterOrder=1  InputFilterTimeConstant=0.001  UdotUserProvided=0
  Sum : Sum  Inputs=-|+
      settings: AttributesFormatString=Error
  Steering Torque : PMIOPort  Port=1  Side=Right
  wires:
  PD Controller Gain/1 -> Simulink-PS Converter/1
  Measured Delta/1 -> Sum/2
  Mux/1 -> PD Controller Gain/1
  Sum/1 -> Mux/1
  Measured DeltaDot/1 -> Mux/2
  Desired Steering Input/1 -> Sum/1
  connections:
  Simulink-PS Converter/RConn1 -- Steering Torque/RConn1

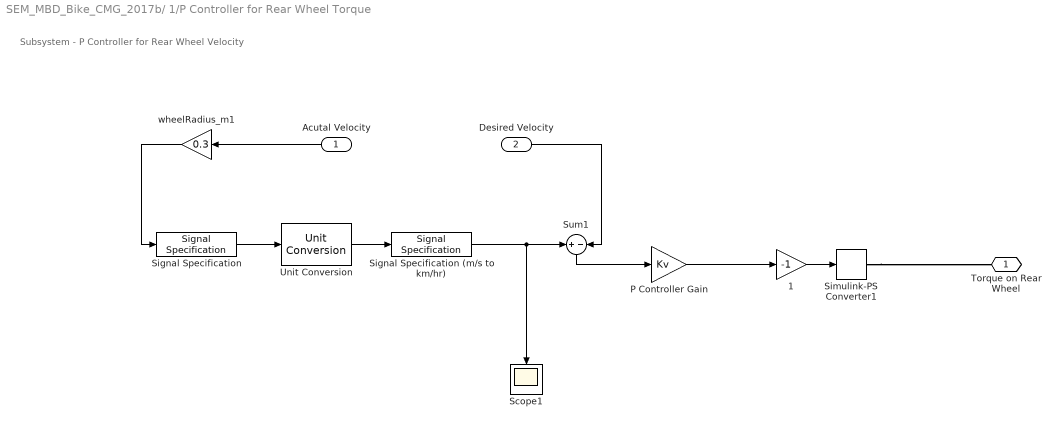
== system SEM_MBD_Bike_CMG_2017b/ 1/P Controller for Rear Wheel Torque  ==
  note: Subsystem - P Controller for Rear Wheel Velocity
  Acutal Velocity : Inport
  Desired Velocity : Inport  Port=2
  1 : Gain  Gain=-1
  P Controller Gain : Gain  Gain=Kv
  Scope1 : Scope
  "Signal Specification " : SignalSpecification  Unit=m/s
  Signal Specification (m/s to km/hr) : SignalSpecification  Unit=km/hr
  Simulink-PS Converter1 : nesl_utility/Simulink-PS Converter  PhysicalDomain=network_engine_domain  SubClassName=ps_input  LeftPortType=input  RightPortType=output  PseudoPeriodic=off  Frequencies=[]  NoiseDistribution=none  NoiseParameters=[]  Unit=N*m  AffineConversion=off  FilteringAndDerivatives=filter  SimscapeFilterOrder=2  InputFilterTimeConstant=1  UdotUserProvided=0
  Sum1 : Sum  Inputs=+|-
  "Unit Conversion " : UnitConversion
  wheelRadius_m1 : Gain  Gain=0.3
      settings: AttributesFormatString=%<Gain>
  Torque on Rear Wheel : PMIOPort  Port=1  Side=Right
  wires:
  Desired Velocity/1 -> Sum1/2
  1/1 -> Simulink-PS Converter1/1
  Acutal Velocity/1 -> wheelRadius_m1/1
  "Unit Conversion "/1 -> Signal Specification (m/s to km/hr)/1
  P Controller Gain/1 -> 1/1
  Signal Specification (m/s to km/hr)/1 -> Scope1/1, Sum1/1
  Sum1/1 -> P Controller Gain/1
  "Signal Specification "/1 -> "Unit Conversion "/1
  wheelRadius_m1/1 -> "Signal Specification "/1
  connections:
  Simulink-PS Converter1/RConn1 -- Torque on Rear Wheel/RConn1

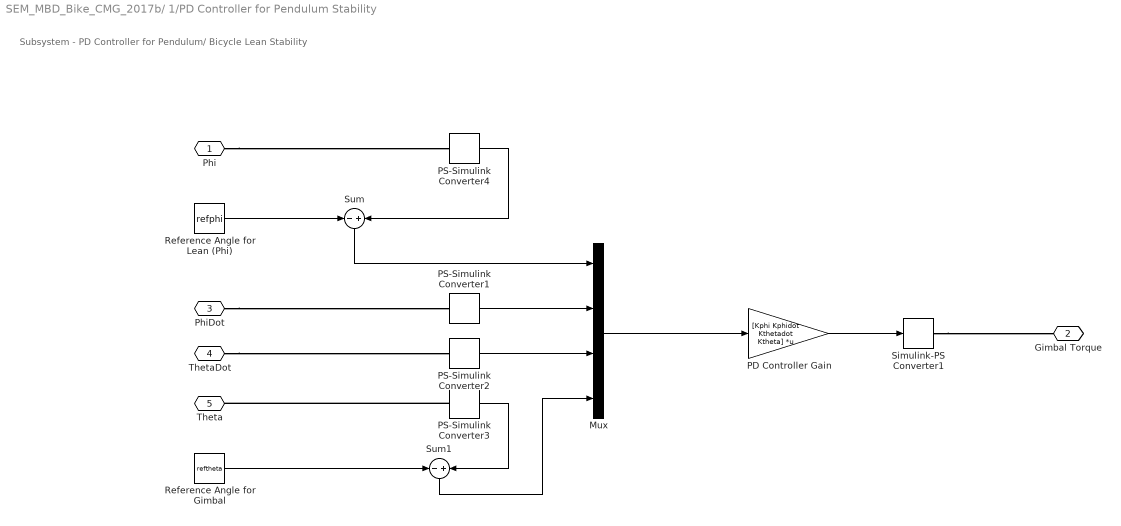
== system SEM_MBD_Bike_CMG_2017b/ 1/PD Controller for Pendulum Stability  ==
  note: Subsystem - PD Controller for Pendulum/ Bicycle Lean Stability
  Mux : Mux
  PD Controller Gain : Gain  Gain=[Kphi Kphidot Kthetadot Ktheta]  Multiplication=Matrix(K*u)
  PS-Simulink Converter{1..4} (4 alike) : nesl_utility/PS-Simulink Converter  PhysicalDomain=network_engine_domain  SubClassName=ps_output  LeftPortType=input  RightPortType=output  PseudoPeriodic=off  Frequencies=[]  Unit=1  AffineConversion=off
  Reference Angle for Gimbal : Constant  Value=reftheta
  Reference Angle for Lean (Phi) : Constant  Value=refphi
  Simulink-PS Converter1 : nesl_utility/Simulink-PS Converter  PhysicalDomain=network_engine_domain  SubClassName=ps_input  LeftPortType=input  RightPortType=output  PseudoPeriodic=off  Frequencies=[]  NoiseDistribution=none  NoiseParameters=[]  Unit=N*m  AffineConversion=off  FilteringAndDerivatives=provide  SimscapeFilterOrder=1  InputFilterTimeConstant=0.001  UdotUserProvided=0
  Sum : Sum  Inputs=-|+
      settings: AttributesFormatString=Error
  Sum1 : Sum  Inputs=-|+
      settings: AttributesFormatString=Error
  Phi : PMIOPort  Port=1  Side=Left
  Gimbal Torque : PMIOPort  Port=2  Side=Right
  PhiDot : PMIOPort  Port=3  Side=Left
  ThetaDot : PMIOPort  Port=4  Side=Left
  Theta : PMIOPort  Port=5  Side=Left
  wires:
  PS-Simulink Converter4/1 -> Sum/2
  Sum1/1 -> Mux/4
  PS-Simulink Converter3/1 -> Sum1/2
  Reference Angle for Gimbal/1 -> Sum1/1
  PS-Simulink Converter2/1 -> Mux/3
  PD Controller Gain/1 -> Simulink-PS Converter1/1
  Mux/1 -> PD Controller Gain/1
  PS-Simulink Converter1/1 -> Mux/2
  Sum/1 -> Mux/1
  Reference Angle for Lean (Phi)/1 -> Sum/1
  connections:
  PS-Simulink Converter3/LConn1 -- Theta/RConn1
  Simulink-PS Converter1/RConn1 -- Gimbal Torque/RConn1
  ThetaDot/RConn1 -- PS-Simulink Converter2/LConn1
  PhiDot/RConn1 -- PS-Simulink Converter1/LConn1
  Phi/RConn1 -- PS-Simulink Converter4/LConn1

== system SEM_MBD_Bike_CMG_2017b/ 1/PD Controller for Steering  ==
  note: Subsystem - PD Controller for Bicycle Steering
  Measured Delta : Inport
  Measured DeltaDot : Inport  Port=2
  Desired Steering Input : Inport  Port=3
  Mux : Mux  Inputs=2
  PD Controller Gain : Gain  Gain=[Kdelta Kdeltadot]  Multiplication=Matrix(K*u)
  Simulink-PS Converter : nesl_utility/Simulink-PS Converter  PhysicalDomain=network_engine_domain  SubClassName=ps_input  LeftPortType=input  RightPortType=output  PseudoPeriodic=off  Frequencies=[]  NoiseDistribution=none  NoiseParameters=[]  Unit=1  AffineConversion=off  FilteringAndDerivatives=provide  SimscapeFilterOrder=1  InputFilterTimeConstant=0.001  UdotUserProvided=0
  Sum : Sum  Inputs=-|+
      settings: AttributesFormatString=Error
  Steering Torque : PMIOPort  Port=1  Side=Right
  wires:
  Desired Steering Input/1 -> Sum/1
  Measured DeltaDot/1 -> Mux/2
  Sum/1 -> Mux/1
  Mux/1 -> PD Controller Gain/1
  Measured Delta/1 -> Sum/2
  PD Controller Gain/1 -> Simulink-PS Converter/1
  connections:
  Simulink-PS Converter/RConn1 -- Steering Torque/RConn1

== system SEM_MBD_Bike_CMG_2017b/           /  Floor ==
  note: Subsystem - Floor
  Grid : Subsystem
  Plane : sm_lib/Body Elements/Solid  InertiaType=CalculateFromGeometry  Mass=1  MassUnits=kg  CenterOfMass=[0 0 0]  CenterOfMassUnits=m  MomentsOfInertia=[1 1 1]  MomentsOfInertiaUnits=kg*m^2  ProductsOfInertia=[0 0 0]  ProductsOfInertiaUnits=kg*m^2  DensityBased=on  Density=1000  DensityUnits=kg/(m^3)  DoExposeReferenceFrame=on  SerializedFrames=<Frames/>  GraphicType=FromGeometry  MarkerShape=Sphere  MarkerSize=10  MarkerSizeUnits=m  GraphicVisPropType=SimpleVisualProperties  GraphicDiffuseColor=[0.8 0.8 0.8]  GraphicSpecularColor=[0.5 0.5 0.5 1.0]  GraphicAmbientColor=[0.15 0.15 0.15 1.0]  GraphicEmissiveColor=[0.0 0.0 0.0 1.0]  GraphicShininess=75  GraphicOpacity=0.5  GeometryShape=Brick  RectangleSize=[1 1]  RectangleSizeUnits=m  BrickDimensions=[Floor.l Floor.w Floor.h]  BrickDimensionUnits=m  CylinderRadius=1  CylinderRadiusUnits=m  CylinderLength=1  CylinderLengthUnits=m  SphereRadius=1  SphereRadiusUnits=m  EllipsoidRadii=[1 1 1]  EllipsoidRadiiUnits=m  ExtrusionCrossSection=[1 1; -1 1; -1 -1; 1 -1]  ExtrusionCrossSectionUnits=m  ExtrusionLength=1  ExtrusionLengthUnits=m  PolygonNumSides=3  PolygonOuterRadius=1  PolygonOuterRadiusUnits=m  ExtGeomFileType=STL  ExtGeomFileUnits=m  RevolutionCrossSection=[1 1; 1 -1; 2 -1; 2 1]  RevolutionCrossSectionUnits=m  RevolutionExtent=Full  RevolutionAngle=180  RevolutionAngleUnits=deg
  B : PMIOPort  Port=1  Side=Right
  F : PMIOPort  Port=2  Side=Left
  connections:
  Plane/RConn1 -- Grid/LConn1 -- F/RConn1 -- B/RConn1
